simulink model "controlSystemDiagrams"  (R2017a)
settings: Solver=VariableStepAuto  StartTime=0.0  StopTime=10.0  RelTol=1e-3
settings Model: Creator=kando  LastModifiedBy=kando

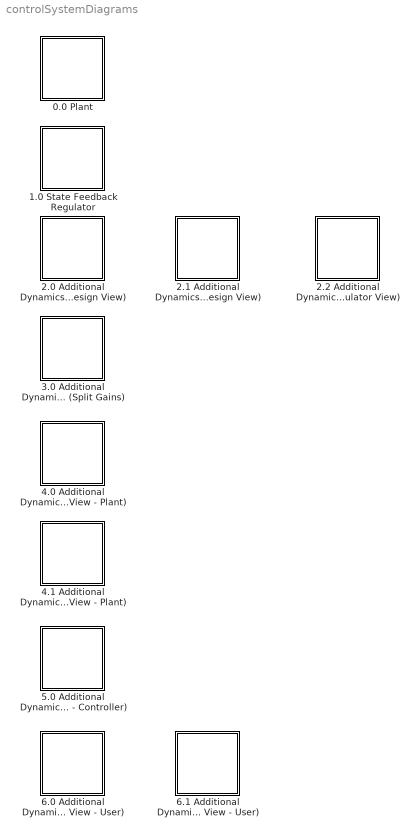
== system controlSystemDiagrams ==
  0.0 Plant : Subsystem
  1.0 State Feedback Regulator : Subsystem
  2.0 Additional Dynamics (Design View) : Subsystem
  2.1 Additional Dynamics (Design View) : Subsystem
  2.2 Additional Dynamics (State Feedback Regulator View) : Subsystem
  3.0 Additional Dynamics (Split Gains) : Subsystem
  4.0 Additional Dynamics (Linear View - Plant) : Subsystem
  4.1 Additional Dynamics (Linear View - Plant) : Subsystem
  5.0 Additional Dynamics (Linear View - Controller) : Subsystem
  6.0 Additional Dynamics (Linear View - User) : Subsystem
  6.1 Additional Dynamics (Linear View - User) : Subsystem

== system controlSystemDiagrams/0.0 Plant ==
  Hardware Dynamics: State-Space Representation Continuous : StateSpace  A=zeros(6,6)  B=zeros(6,2)  C=eye(6,6)  D=zeros(6,2)  X0=zeros(6,1)
      settings: AttributesFormatString=|
      | C = %<C>
      | D = %<D>

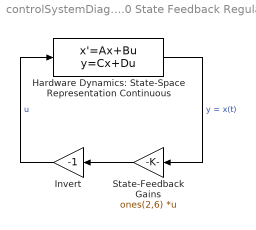
== system controlSystemDiagrams/1.0 State Feedback Regulator ==
  Hardware Dynamics: State-Space Representation Continuous : StateSpace  A=zeros(6,6)  B=zeros(6,2)  C=eye(6,6)  D=zeros(6,2)  X0=zeros(6,1)
      settings: AttributesFormatString=|
      | C = %<C>
      | D = %<D>
  Invert : Gain  Gain=-1
  State-Feedback Gains : Gain  Gain=ones(2,6)  Multiplication=Matrix(K*u)
  wires:
  Invert/1 -> Hardware Dynamics: State-Space Representation Continuous/1  "u"
  State-Feedback Gains/1 -> Invert/1
  Hardware Dynamics: State-Space Representation Continuous/1 -> State-Feedback Gains/1  "y = x(t)"

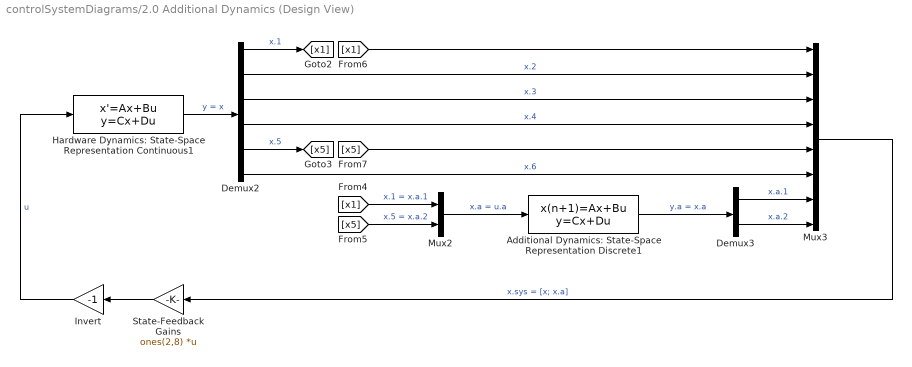
== system controlSystemDiagrams/2.0 Additional Dynamics (Design View) ==
  Additional Dynamics: State-Space Representation Discrete1 : DiscreteStateSpace  A=zeros(2,2)  B=eye(2,2)  C=eye(2,2)  D=zeros(2,2)  X0=zeros(2,1)  SampleTime=-1
      settings: AttributesFormatString=|
      | C.a = %<C>
      | D.a = %<D>
  Demux2 : Demux  Outputs=6
  Demux3 : Demux  Outputs=2
  Hardware Dynamics: State-Space Representation Continuous1 : StateSpace  A=zeros(6,6)  B=zeros(6,2)  C=eye(6,6)  D=zeros(6,2)  X0=zeros(6,1)
      settings: AttributesFormatString=|
      | C = %<C>
      | D = %<D>
  Invert : Gain  Gain=-1
  Mux2 : Mux  Inputs=2
  Mux3 : Mux  Inputs=8
  State-Feedback Gains : Gain  Gain=ones(2,8)  Multiplication=Matrix(K*u)
  wires:
  State-Feedback Gains/1 -> Invert/1
  Mux2/1 -> Additional Dynamics: State-Space Representation Discrete1/1  "x.a = u.a"
  Demux2/5 -> [x5]  "x.5"
  Invert/1 -> Hardware Dynamics: State-Space Representation Continuous1/1  "u"
  [x5] -> Mux3/5
  Mux3/1 -> State-Feedback Gains/1  "x.sys = [x; x.a]"
  [x5] -> Mux2/2  "x.5 = x.a.2"
  Hardware Dynamics: State-Space Representation Continuous1/1 -> Demux2/1  "y = x"
  Demux2/1 -> [x1]  "x.1"
  Additional Dynamics: State-Space Representation Discrete1/1 -> Demux3/1  "y.a = x.a"
  Demux2/3 -> Mux3/3  "x.3"
  Demux3/2 -> Mux3/8  "x.a.2"
  Demux2/4 -> Mux3/4  "x.4"
  Demux2/2 -> Mux3/2  "x.2"
  Demux3/1 -> Mux3/7  "x.a.1"
  [x1] -> Mux3/1
  Demux2/6 -> Mux3/6  "x.6"
  [x1] -> Mux2/1  "x.1 = x.a.1"

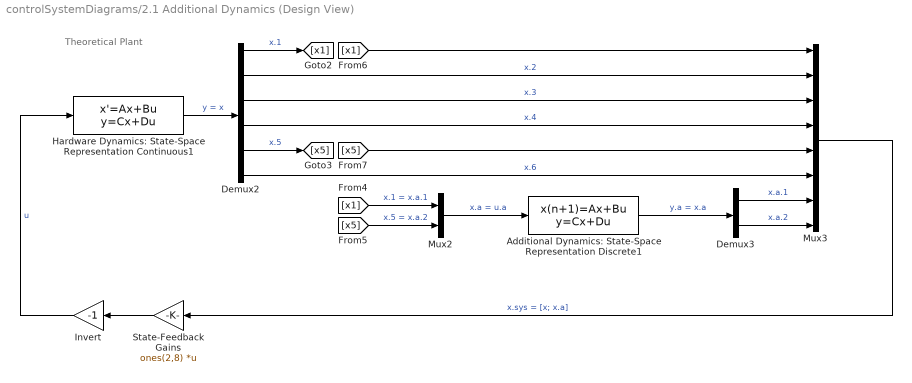
== system controlSystemDiagrams/2.1 Additional Dynamics (Design View) ==
  note: Theoretical Plant
  Additional Dynamics: State-Space Representation Discrete1 : DiscreteStateSpace  A=zeros(2,2)  B=eye(2,2)  C=eye(2,2)  D=zeros(2,2)  X0=zeros(2,1)  SampleTime=-1
      settings: AttributesFormatString=|
      | C.a = %<C>
      | D.a = %<D>
  Demux2 : Demux  Outputs=6
  Demux3 : Demux  Outputs=2
  Hardware Dynamics: State-Space Representation Continuous1 : StateSpace  A=zeros(6,6)  B=zeros(6,2)  C=eye(6,6)  D=zeros(6,2)  X0=zeros(6,1)
      settings: AttributesFormatString=|
      | C = %<C>
      | D = %<D>
  Invert : Gain  Gain=-1
  Mux2 : Mux  Inputs=2
  Mux3 : Mux  Inputs=8
  State-Feedback Gains : Gain  Gain=ones(2,8)  Multiplication=Matrix(K*u)
  wires:
  [x1] -> Mux2/1  "x.1 = x.a.1"
  Demux2/6 -> Mux3/6  "x.6"
  [x1] -> Mux3/1
  Demux3/1 -> Mux3/7  "x.a.1"
  Demux2/2 -> Mux3/2  "x.2"
  Demux2/4 -> Mux3/4  "x.4"
  Demux3/2 -> Mux3/8  "x.a.2"
  Demux2/3 -> Mux3/3  "x.3"
  Additional Dynamics: State-Space Representation Discrete1/1 -> Demux3/1  "y.a = x.a"
  Demux2/1 -> [x1]  "x.1"
  Hardware Dynamics: State-Space Representation Continuous1/1 -> Demux2/1  "y = x"
  [x5] -> Mux2/2  "x.5 = x.a.2"
  Mux3/1 -> State-Feedback Gains/1  "x.sys = [x; x.a]"
  [x5] -> Mux3/5
  Invert/1 -> Hardware Dynamics: State-Space Representation Continuous1/1  "u"
  Demux2/5 -> [x5]  "x.5"
  Mux2/1 -> Additional Dynamics: State-Space Representation Discrete1/1  "x.a = u.a"
  State-Feedback Gains/1 -> Invert/1

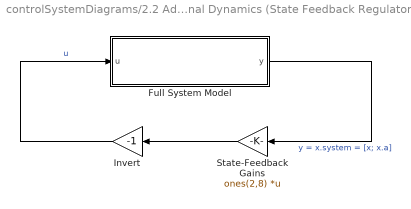
== system controlSystemDiagrams/2.2 Additional Dynamics (State Feedback Regulator View) ==
  Full System Model : Subsystem
  Invert : Gain  Gain=-1
  State-Feedback Gains : Gain  Gain=ones(2,8)  Multiplication=Matrix(K*u)
  wires:
  Full System Model/1(y) -> State-Feedback Gains/1  "y = x.system = [x; x.a]"
  State-Feedback Gains/1 -> Invert/1
  Invert/1 -> Full System Model/1(u)  "u"

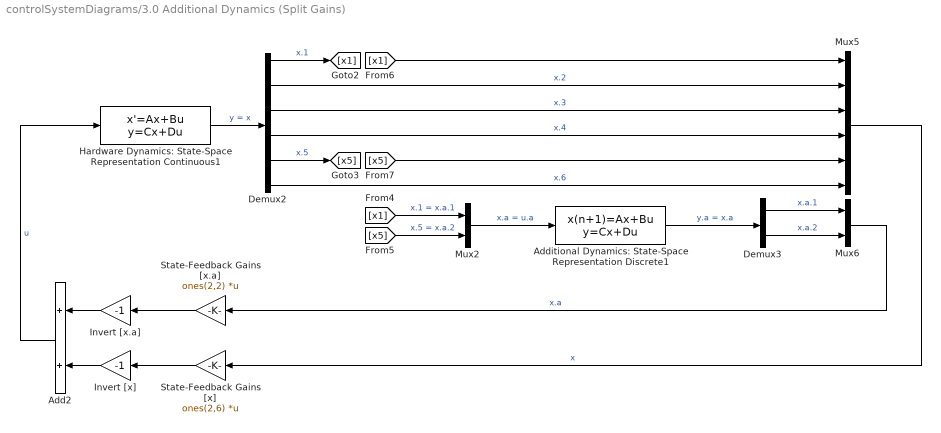
== system controlSystemDiagrams/3.0 Additional Dynamics (Split Gains) ==
  Add2 : Sum
  Additional Dynamics: State-Space Representation Discrete1 : DiscreteStateSpace  A=zeros(2,2)  B=eye(2,2)  C=eye(2,2)  D=zeros(2,2)  X0=zeros(2,1)  SampleTime=-1
      settings: AttributesFormatString=|
      | C.a = %<C>
      | D.a = %<D>
  Demux2 : Demux  Outputs=6
  Demux3 : Demux  Outputs=2
  Hardware Dynamics: State-Space Representation Continuous1 : StateSpace  A=zeros(6,6)  B=zeros(6,2)  C=eye(6,6)  D=zeros(6,2)  X0=zeros(6,1)
      settings: AttributesFormatString=|
      | C = %<C>
      | D = %<D>
  Invert [x.a] : Gain  Gain=-1
  Invert [x] : Gain  Gain=-1
  Mux2 : Mux  Inputs=2
  Mux5 : Mux  Inputs=6
  Mux6 : Mux  Inputs=2
  State-Feedback Gains [x.a] : Gain  Gain=ones(2,2)  Multiplication=Matrix(K*u)
  State-Feedback Gains [x] : Gain  Gain=ones(2,6)  Multiplication=Matrix(K*u)
  wires:
  State-Feedback Gains [x.a]/1 -> Invert [x.a]/1
  Invert [x]/1 -> Add2/2
  Mux5/1 -> State-Feedback Gains [x]/1  "x"
  State-Feedback Gains [x]/1 -> Invert [x]/1
  Invert [x.a]/1 -> Add2/1
  Mux6/1 -> State-Feedback Gains [x.a]/1  "x.a"
  Add2/1 -> Hardware Dynamics: State-Space Representation Continuous1/1  "u"
  [x5] -> Mux5/5
  Demux2/2 -> Mux5/2  "x.2"
  Demux2/3 -> Mux5/3  "x.3"
  Demux3/2 -> Mux6/2  "x.a.2"
  Demux2/6 -> Mux5/6  "x.6"
  Demux3/1 -> Mux6/1  "x.a.1"
  Demux2/1 -> [x1]  "x.1"
  Demux2/4 -> Mux5/4  "x.4"
  Demux2/5 -> [x5]  "x.5"
  Additional Dynamics: State-Space Representation Discrete1/1 -> Demux3/1  "y.a = x.a"
  [x1] -> Mux2/1  "x.1 = x.a.1"
  [x5] -> Mux2/2  "x.5 = x.a.2"
  Mux2/1 -> Additional Dynamics: State-Space Representation Discrete1/1  "x.a = u.a"
  Hardware Dynamics: State-Space Representation Continuous1/1 -> Demux2/1  "y = x"
  [x1] -> Mux5/1

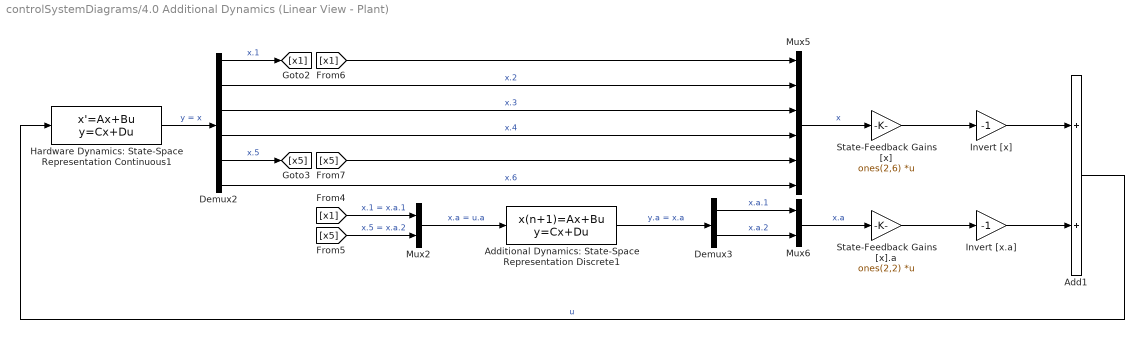
== system controlSystemDiagrams/4.0 Additional Dynamics (Linear View - Plant) ==
  Add1 : Sum
  Additional Dynamics: State-Space Representation Discrete1 : DiscreteStateSpace  A=zeros(2,2)  B=eye(2,2)  C=eye(2,2)  D=zeros(2,2)  X0=zeros(2,1)  SampleTime=-1
      settings: AttributesFormatString=|
      | C.a = %<C>
      | D.a = %<D>
  Demux2 : Demux  Outputs=6
  Demux3 : Demux  Outputs=2
  Hardware Dynamics: State-Space Representation Continuous1 : StateSpace  A=zeros(6,6)  B=zeros(6,2)  C=eye(6,6)  D=zeros(6,2)  X0=zeros(6,1)
      settings: AttributesFormatString=|
      | C = %<C>
      | D = %<D>
  Invert [x.a] : Gain  Gain=-1
  Invert [x] : Gain  Gain=-1
  Mux2 : Mux  Inputs=2
  Mux5 : Mux  Inputs=6
  Mux6 : Mux  Inputs=2
  State-Feedback Gains [x] : Gain  Gain=ones(2,6)  Multiplication=Matrix(K*u)
  State-Feedback Gains [x].a : Gain  Gain=ones(2,2)  Multiplication=Matrix(K*u)
  wires:
  Mux6/1 -> State-Feedback Gains [x].a/1  "x.a"
  State-Feedback Gains [x].a/1 -> Invert [x.a]/1
  Add1/1 -> Hardware Dynamics: State-Space Representation Continuous1/1  "u"
  State-Feedback Gains [x]/1 -> Invert [x]/1
  Mux5/1 -> State-Feedback Gains [x]/1  "x"
  Invert [x]/1 -> Add1/1
  Invert [x.a]/1 -> Add1/2
  [x1] -> Mux5/1
  Hardware Dynamics: State-Space Representation Continuous1/1 -> Demux2/1  "y = x"
  Demux3/1 -> Mux6/1  "x.a.1"
  Demux2/3 -> Mux5/3  "x.3"
  [x5] -> Mux2/2  "x.5 = x.a.2"
  Demux3/2 -> Mux6/2  "x.a.2"
  Demux2/5 -> [x5]  "x.5"
  Mux2/1 -> Additional Dynamics: State-Space Representation Discrete1/1  "x.a = u.a"
  Demux2/4 -> Mux5/4  "x.4"
  [x5] -> Mux5/5
  [x1] -> Mux2/1  "x.1 = x.a.1"
  Demux2/2 -> Mux5/2  "x.2"
  Additional Dynamics: State-Space Representation Discrete1/1 -> Demux3/1  "y.a = x.a"
  Demux2/1 -> [x1]  "x.1"
  Demux2/6 -> Mux5/6  "x.6"

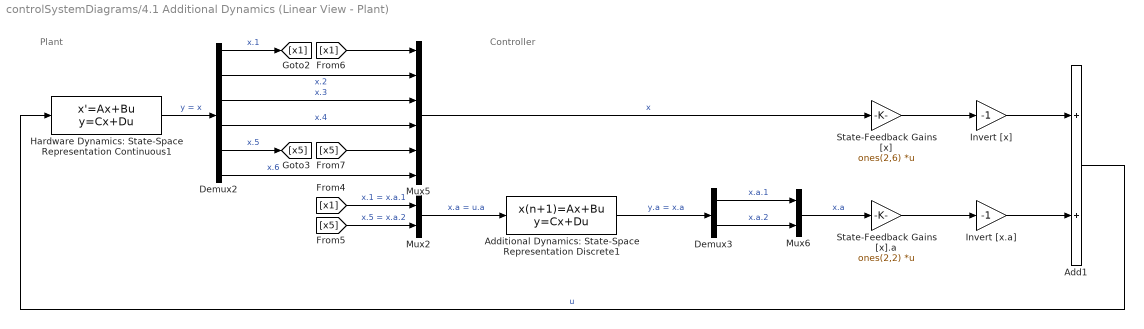
== system controlSystemDiagrams/4.1 Additional Dynamics (Linear View - Plant) ==
  note: Plant
  note: Controller
  Add1 : Sum
  Additional Dynamics: State-Space Representation Discrete1 : DiscreteStateSpace  A=zeros(2,2)  B=eye(2,2)  C=eye(2,2)  D=zeros(2,2)  X0=zeros(2,1)  SampleTime=-1
      settings: AttributesFormatString=|
      | C.a = %<C>
      | D.a = %<D>
  Demux2 : Demux  Outputs=6
  Demux3 : Demux  Outputs=2
  Hardware Dynamics: State-Space Representation Continuous1 : StateSpace  A=zeros(6,6)  B=zeros(6,2)  C=eye(6,6)  D=zeros(6,2)  X0=zeros(6,1)
      settings: AttributesFormatString=|
      | C = %<C>
      | D = %<D>
  Invert [x.a] : Gain  Gain=-1
  Invert [x] : Gain  Gain=-1
  Mux2 : Mux  Inputs=2
  Mux5 : Mux  Inputs=6
  Mux6 : Mux  Inputs=2
  State-Feedback Gains [x] : Gain  Gain=ones(2,6)  Multiplication=Matrix(K*u)
  State-Feedback Gains [x].a : Gain  Gain=ones(2,2)  Multiplication=Matrix(K*u)
  wires:
  Demux2/6 -> Mux5/6  "x.6"
  Demux2/1 -> [x1]  "x.1"
  Additional Dynamics: State-Space Representation Discrete1/1 -> Demux3/1  "y.a = x.a"
  Demux2/2 -> Mux5/2  "x.2"
  [x1] -> Mux2/1  "x.1 = x.a.1"
  [x5] -> Mux5/5
  Demux2/4 -> Mux5/4  "x.4"
  Mux2/1 -> Additional Dynamics: State-Space Representation Discrete1/1  "x.a = u.a"
  Demux2/5 -> [x5]  "x.5"
  Demux3/2 -> Mux6/2  "x.a.2"
  [x5] -> Mux2/2  "x.5 = x.a.2"
  Demux2/3 -> Mux5/3  "x.3"
  Demux3/1 -> Mux6/1  "x.a.1"
  Hardware Dynamics: State-Space Representation Continuous1/1 -> Demux2/1  "y = x"
  [x1] -> Mux5/1
  Invert [x.a]/1 -> Add1/2
  Invert [x]/1 -> Add1/1
  Mux5/1 -> State-Feedback Gains [x]/1  "x"
  State-Feedback Gains [x]/1 -> Invert [x]/1
  Add1/1 -> Hardware Dynamics: State-Space Representation Continuous1/1  "u"
  State-Feedback Gains [x].a/1 -> Invert [x.a]/1
  Mux6/1 -> State-Feedback Gains [x].a/1  "x.a"

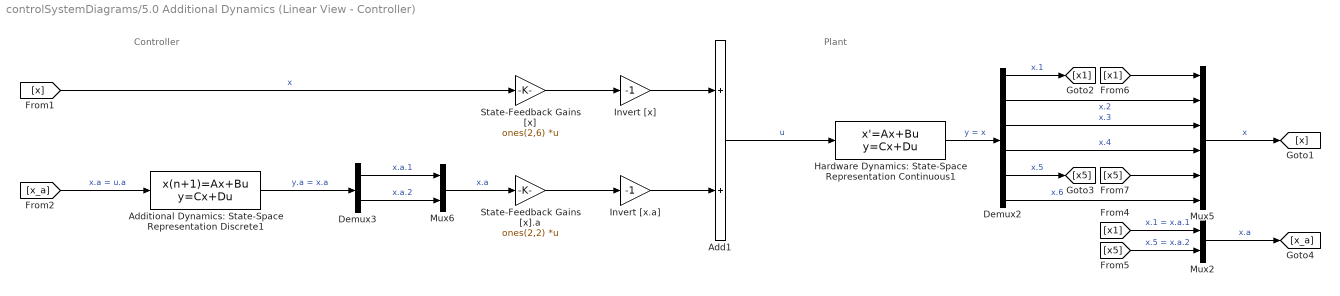
== system controlSystemDiagrams/5.0 Additional Dynamics (Linear View - Controller) ==
  note: Plant
  note: Controller
  Add1 : Sum
  Additional Dynamics: State-Space Representation Discrete1 : DiscreteStateSpace  A=zeros(2,2)  B=eye(2,2)  C=eye(2,2)  D=zeros(2,2)  X0=zeros(2,1)  SampleTime=-1
      settings: AttributesFormatString=|
      | C.a = %<C>
      | D.a = %<D>
  Demux2 : Demux  Outputs=6
  Demux3 : Demux  Outputs=2
  Hardware Dynamics: State-Space Representation Continuous1 : StateSpace  A=zeros(6,6)  B=zeros(6,2)  C=eye(6,6)  D=zeros(6,2)  X0=zeros(6,1)
      settings: AttributesFormatString=|
      | C = %<C>
      | D = %<D>
  Invert [x.a] : Gain  Gain=-1
  Invert [x] : Gain  Gain=-1
  Mux2 : Mux  Inputs=2
  Mux5 : Mux  Inputs=6
  Mux6 : Mux  Inputs=2
  State-Feedback Gains [x] : Gain  Gain=ones(2,6)  Multiplication=Matrix(K*u)
  State-Feedback Gains [x].a : Gain  Gain=ones(2,2)  Multiplication=Matrix(K*u)
  wires:
  Demux2/1 -> [x1]  "x.1"
  Demux2/4 -> Mux5/4  "x.4"
  [x5] -> Mux2/2  "x.5 = x.a.2"
  Invert [x]/1 -> Add1/1
  Demux2/6 -> Mux5/6  "x.6"
  Demux3/1 -> Mux6/1  "x.a.1"
  Mux5/1 -> [x]  "x"
  Mux2/1 -> [x_a]  "x.a"
  [x1] -> Mux2/1  "x.1 = x.a.1"
  Additional Dynamics: State-Space Representation Discrete1/1 -> Demux3/1  "y.a = x.a"
  Invert [x.a]/1 -> Add1/2
  Mux6/1 -> State-Feedback Gains [x].a/1  "x.a"
  Demux3/2 -> Mux6/2  "x.a.2"
  State-Feedback Gains [x].a/1 -> Invert [x.a]/1
  Hardware Dynamics: State-Space Representation Continuous1/1 -> Demux2/1  "y = x"
  Demux2/2 -> Mux5/2  "x.2"
  [x1] -> Mux5/1
  State-Feedback Gains [x]/1 -> Invert [x]/1
  Demux2/5 -> [x5]  "x.5"
  Add1/1 -> Hardware Dynamics: State-Space Representation Continuous1/1  "u"
  Demux2/3 -> Mux5/3  "x.3"
  [x5] -> Mux5/5
  [x] -> State-Feedback Gains [x]/1  "x"
  [x_a] -> Additional Dynamics: State-Space Representation Discrete1/1  "x.a = u.a"

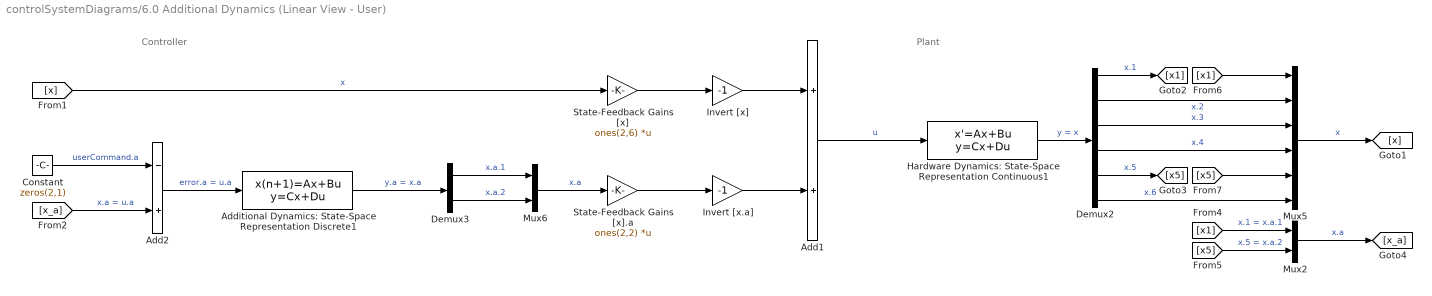
== system controlSystemDiagrams/6.0 Additional Dynamics (Linear View - User) ==
  note: Controller
  note: Plant
  Add1 : Sum
  Add2 : Sum  Inputs=-+
  Additional Dynamics: State-Space Representation Discrete1 : DiscreteStateSpace  A=zeros(2,2)  B=eye(2,2)  C=eye(2,2)  D=zeros(2,2)  X0=zeros(2,1)  SampleTime=-1
      settings: AttributesFormatString=|
      | C.a = %<C>
      | D.a = %<D>
  Constant : Constant  Value=zeros(2,1)
      settings: AttributesFormatString=%<Value>
  Demux2 : Demux  Outputs=6
  Demux3 : Demux  Outputs=2
  Hardware Dynamics: State-Space Representation Continuous1 : StateSpace  A=zeros(6,6)  B=zeros(6,2)  C=eye(6,6)  D=zeros(6,2)  X0=zeros(6,1)
      settings: AttributesFormatString=|
      | C = %<C>
      | D = %<D>
  Invert [x.a] : Gain  Gain=-1
  Invert [x] : Gain  Gain=-1
  Mux2 : Mux  Inputs=2
  Mux5 : Mux  Inputs=6
  Mux6 : Mux  Inputs=2
  State-Feedback Gains [x] : Gain  Gain=ones(2,6)  Multiplication=Matrix(K*u)
  State-Feedback Gains [x].a : Gain  Gain=ones(2,2)  Multiplication=Matrix(K*u)
  wires:
  State-Feedback Gains [x]/1 -> Invert [x]/1
  [x] -> State-Feedback Gains [x]/1  "x"
  Add2/1 -> Additional Dynamics: State-Space Representation Discrete1/1  "error.a = u.a"
  Demux2/2 -> Mux5/2  "x.2"
  State-Feedback Gains [x].a/1 -> Invert [x.a]/1
  Mux2/1 -> [x_a]  "x.a"
  Invert [x]/1 -> Add1/1
  [x1] -> Mux5/1
  Demux2/4 -> Mux5/4  "x.4"
  Demux2/5 -> [x5]  "x.5"
  Demux2/6 -> Mux5/6  "x.6"
  [x5] -> Mux5/5
  Hardware Dynamics: State-Space Representation Continuous1/1 -> Demux2/1  "y = x"
  [x5] -> Mux2/2  "x.5 = x.a.2"
  Additional Dynamics: State-Space Representation Discrete1/1 -> Demux3/1  "y.a = x.a"
  Invert [x.a]/1 -> Add1/2
  Demux3/2 -> Mux6/2  "x.a.2"
  Demux2/3 -> Mux5/3  "x.3"
  Demux3/1 -> Mux6/1  "x.a.1"
  [x1] -> Mux2/1  "x.1 = x.a.1"
  Mux5/1 -> [x]  "x"
  Add1/1 -> Hardware Dynamics: State-Space Representation Continuous1/1  "u"
  Demux2/1 -> [x1]  "x.1"
  Mux6/1 -> State-Feedback Gains [x].a/1  "x.a"
  [x_a] -> Add2/2  "x.a = u.a"
  Constant/1 -> Add2/1  "userCommand.a"

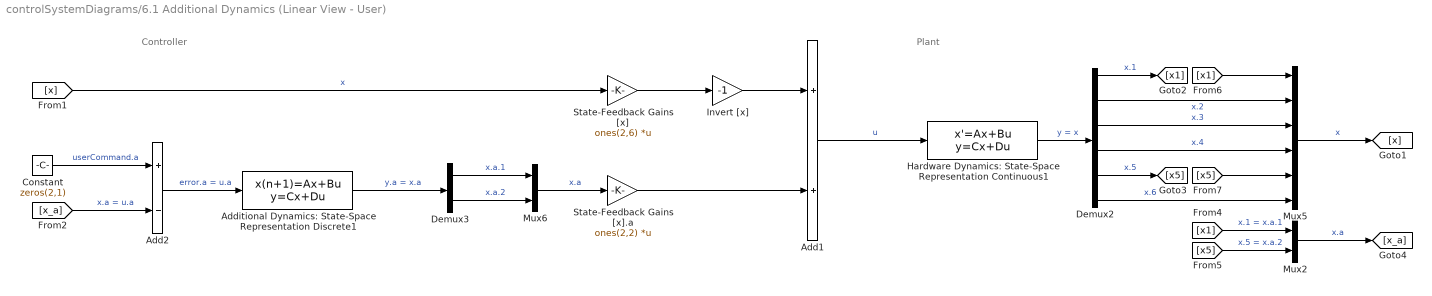
== system controlSystemDiagrams/6.1 Additional Dynamics (Linear View - User) ==
  note: Controller
  note: Plant
  Add1 : Sum
  Add2 : Sum  Inputs=+-
  Additional Dynamics: State-Space Representation Discrete1 : DiscreteStateSpace  A=zeros(2,2)  B=eye(2,2)  C=eye(2,2)  D=zeros(2,2)  X0=zeros(2,1)  SampleTime=-1
      settings: AttributesFormatString=|
      | C.a = %<C>
      | D.a = %<D>
  Constant : Constant  Value=zeros(2,1)
      settings: AttributesFormatString=%<Value>
  Demux2 : Demux  Outputs=6
  Demux3 : Demux  Outputs=2
  Hardware Dynamics: State-Space Representation Continuous1 : StateSpace  A=zeros(6,6)  B=zeros(6,2)  C=eye(6,6)  D=zeros(6,2)  X0=zeros(6,1)
      settings: AttributesFormatString=|
      | C = %<C>
      | D = %<D>
  Invert [x] : Gain  Gain=-1
  Mux2 : Mux  Inputs=2
  Mux5 : Mux  Inputs=6
  Mux6 : Mux  Inputs=2
  State-Feedback Gains [x] : Gain  Gain=ones(2,6)  Multiplication=Matrix(K*u)
  State-Feedback Gains [x].a : Gain  Gain=ones(2,2)  Multiplication=Matrix(K*u)
  wires:
  Constant/1 -> Add2/1  "userCommand.a"
  [x5] -> Mux5/5
  Demux2/2 -> Mux5/2  "x.2"
  Demux2/3 -> Mux5/3  "x.3"
  Demux3/2 -> Mux6/2  "x.a.2"
  Demux2/4 -> Mux5/4  "x.4"
  State-Feedback Gains [x]/1 -> Invert [x]/1
  [x_a] -> Add2/2  "x.a = u.a"
  [x5] -> Mux2/2  "x.5 = x.a.2"
  [x1] -> Mux5/1
  Add2/1 -> Additional Dynamics: State-Space Representation Discrete1/1  "error.a = u.a"
  Demux3/1 -> Mux6/1  "x.a.1"
  [x] -> State-Feedback Gains [x]/1  "x"
  State-Feedback Gains [x].a/1 -> Add1/2
  Mux2/1 -> [x_a]  "x.a"
  Hardware Dynamics: State-Space Representation Continuous1/1 -> Demux2/1  "y = x"
  Demux2/1 -> [x1]  "x.1"
  Mux5/1 -> [x]  "x"
  [x1] -> Mux2/1  "x.1 = x.a.1"
  Additional Dynamics: State-Space Representation Discrete1/1 -> Demux3/1  "y.a = x.a"
  Invert [x]/1 -> Add1/1
  Mux6/1 -> State-Feedback Gains [x].a/1  "x.a"
  Demux2/6 -> Mux5/6  "x.6"
  Add1/1 -> Hardware Dynamics: State-Space Representation Continuous1/1  "u"
  Demux2/5 -> [x5]  "x.5"

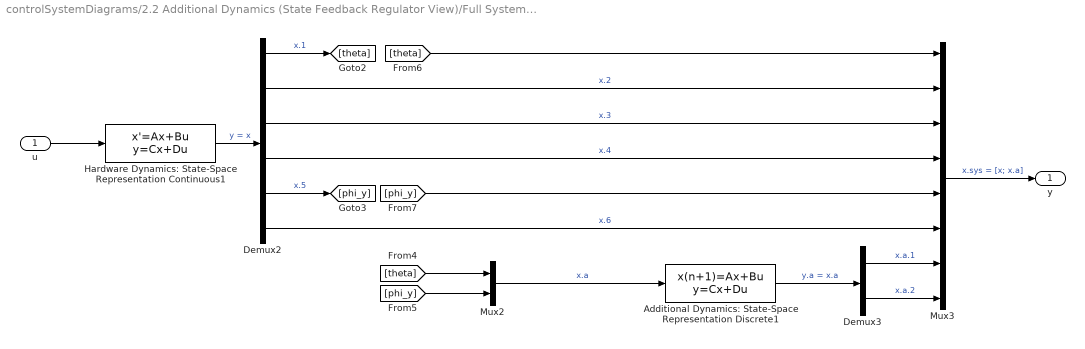
== system controlSystemDiagrams/2.2 Additional Dynamics (State Feedback Regulator View)/Full System Model ==
  u : Inport
  Additional Dynamics: State-Space Representation Discrete1 : DiscreteStateSpace  A=zeros(2,2)  B=eye(2,2)  C=eye(2,2)  D=zeros(2,2)  X0=zeros(2,1)  SampleTime=-1
      settings: AttributesFormatString=|
      | C.a = %<C>
      | D.a = %<D>
  Demux2 : Demux  Outputs=6
  Demux3 : Demux  Outputs=2
  Hardware Dynamics: State-Space Representation Continuous1 : StateSpace  A=zeros(6,6)  B=zeros(6,2)  C=eye(6,6)  D=zeros(6,2)  X0=zeros(6,1)
      settings: AttributesFormatString=|
      | C = %<C>
      | D = %<D>
  Mux2 : Mux  Inputs=2
  Mux3 : Mux  Inputs=8
  y : Outport
  wires:
  u/1 -> Hardware Dynamics: State-Space Representation Continuous1/1
  Demux2/4 -> Mux3/4  "x.4"
  Demux3/1 -> Mux3/7  "x.a.1"
  Mux2/1 -> Additional Dynamics: State-Space Representation Discrete1/1  "x.a"
  [theta] -> Mux2/1
  Hardware Dynamics: State-Space Representation Continuous1/1 -> Demux2/1  "y = x"
  Mux3/1 -> y/1  "x.sys = [x; x.a]"
  Demux2/2 -> Mux3/2  "x.2"
  [phi_y] -> Mux2/2
  Demux3/2 -> Mux3/8  "x.a.2"
  [phi_y] -> Mux3/5
  Additional Dynamics: State-Space Representation Discrete1/1 -> Demux3/1  "y.a = x.a"
  Demux2/1 -> [theta]  "x.1"
  [theta] -> Mux3/1
  Demux2/5 -> [phi_y]  "x.5"
  Demux2/6 -> Mux3/6  "x.6"
  Demux2/3 -> Mux3/3  "x.3"
